simulink model "q_servo_speed_cntrl2"  (R2019a)
settings: Solver=ode4  StartTime=0.0  StopTime=inf  FixedStep=0.002  RelTol=1e-3
values from neighbouring files (symbols this model uses):
  a = 1    [setup_servo_speed_cntrl2.m]
  bsp = 0    [setup_servo_speed_cntrl2.m]
  Kc = 0    [setup_servo_speed_cntrl2.m]
  ki = 0    [setup_servo_speed_cntrl2.m]
  kp = 0    [setup_servo_speed_cntrl2.m]
  T = 1    [setup_servo_speed_cntrl2.m]
undefined symbols (not defined in the file or in its folder): HIL, K_ENC, qc_get_step_size
libraries: quarc_library x6, simulink x2
settings Model: ExtModeTrigDuration=10000  Creator=MLevis  LastModifiedBy=pmartin
settings DataIOCC: ReturnWorkspaceOutputs=off
settings DebuggingCC: UnderspecifiedInitializationDetection=Classic  MergeDetectMultiDrivingBlocksExec=none
settings ModelReferenceCC: PropagateSignalLabelsOutOfModel=off

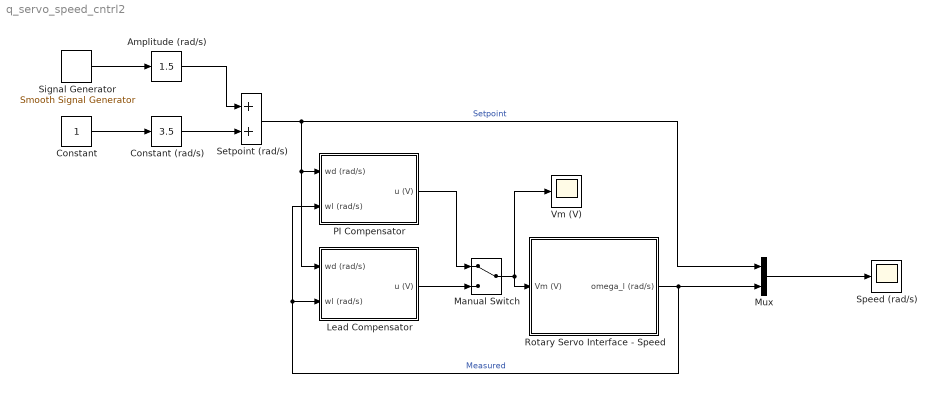
== system q_servo_speed_cntrl2 ==
  Amplitude (rad/s) : simulink/Math Operations/Slider Gain  gain=1.5  low=0  high=10
  "Constant " : Constant
  Constant (rad/s) : simulink/Math Operations/Slider Gain  gain=3.5  low=0  high=10
  Lead Compensator : Subsystem
  Manual Switch : ManualSwitch
  Mux : Mux  Inputs=2
  PI Compensator : Subsystem
  Rotary Servo Interface - Speed : Subsystem
  Setpoint (rad/s) : Sum
  Signal Generator : quarc_library/Sources/Signals/Smooth Signal Generator  signal_type=Square  source=Internal (dialog parameters)  amplitude=1  frequency=0.4  initial_phase=0  sample_time=qc_get_step_size  output_cos=off
      settings: SourceProductName=QUARC Targets
  Speed (rad/s) : Scope
  Vm (V) : Scope
  wires:
  Setpoint (rad/s)/1 -> Mux/1, PI Compensator/1(wd (rad/s)), Lead Compensator/1(wd (rad/s))  "Setpoint"
  Mux/1 -> Speed (rad/s)/1
  Signal Generator/1 -> Amplitude (rad/s)/1
  Amplitude (rad/s)/1 -> Setpoint (rad/s)/1
  "Constant "/1 -> Constant (rad/s)/1
  PI Compensator/1(u (V)) -> Manual Switch/1
  Lead Compensator/1(u (V)) -> Manual Switch/2
  Manual Switch/1 -> Vm (V)/1, Rotary Servo Interface - Speed/1(Vm (V))
  Constant (rad/s)/1 -> Setpoint (rad/s)/2
  Rotary Servo Interface - Speed/1(omega_l (rad/s)) -> Mux/2, Lead Compensator/2(wl (rad/s)), PI Compensator/2(wl (rad/s))  "Measured"

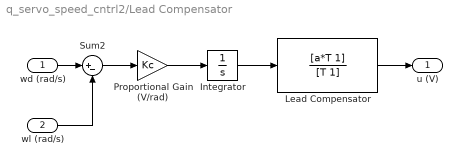
== system q_servo_speed_cntrl2/Lead Compensator ==
  wd (rad/s) : Inport
  wl (rad/s) : Inport  Port=2
  Integrator : Integrator
  Lead Compensator : TransferFcn  Numerator=[a*T 1]  Denominator=[T 1]
  Proportional Gain (V/rad) : Gain  Gain=Kc
  Sum2 : Sum  Inputs=|+-
  u (V) : Outport
  wires:
  wl (rad/s)/1 -> Sum2/2
  wd (rad/s)/1 -> Sum2/1
  Lead Compensator/1 -> u (V)/1
  Sum2/1 -> Proportional Gain (V/rad)/1
  Proportional Gain (V/rad)/1 -> Integrator/1
  Integrator/1 -> Lead Compensator/1

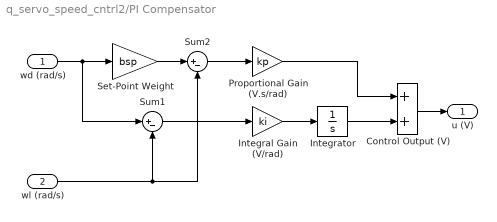
== system q_servo_speed_cntrl2/PI Compensator ==
  wd (rad/s) : Inport
  wl (rad/s) : Inport  Port=2
  Control Output (V) : Sum
  Integral Gain (V/rad) : Gain  Gain=ki
  Integrator : Integrator  UpperSaturationLimit=10  LowerSaturationLimit=-10
  Proportional Gain (V.s/rad) : Gain  Gain=kp
  Set-Point Weight : Gain  Gain=bsp
  Sum1 : Sum  Inputs=|+-
  Sum2 : Sum  Inputs=|+-
  u (V) : Outport
  wires:
  wl (rad/s)/1 -> Sum2/2, Sum1/2
  Control Output (V)/1 -> u (V)/1
  wd (rad/s)/1 -> Sum1/1, Set-Point Weight/1
  Sum2/1 -> Proportional Gain (V.s/rad)/1
  Set-Point Weight/1 -> Sum2/1
  Proportional Gain (V.s/rad)/1 -> Control Output (V)/1
  Integrator/1 -> Control Output (V)/2
  Integral Gain (V/rad)/1 -> Integrator/1
  Sum1/1 -> Integral Gain (V/rad)/1

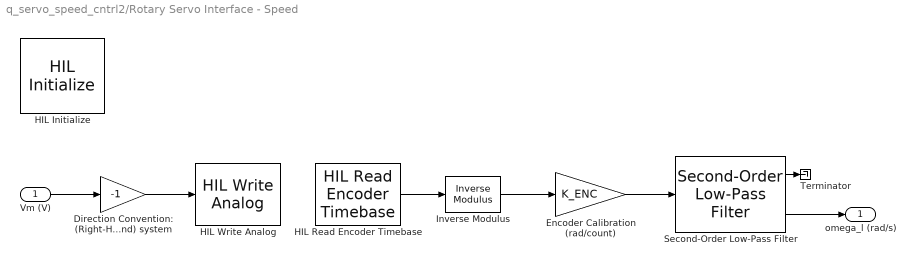
== system q_servo_speed_cntrl2/Rotary Servo Interface - Speed ==
  Vm (V) : Inport
  Direction Convention: (Right-Hand) system : Gain  Gain=-1  SaturateOnIntegerOverflow=on  OutDataTypeStr=Inherit: Same as input  ParamDataTypeStr=Inherit: Same as input
  Encoder Calibration (rad/count) : Gain  Gain=K_ENC  SaturateOnIntegerOverflow=on  OutDataTypeStr=Inherit: Same as input  ParamDataTypeStr=Inherit: Same as input
  HIL Initialize : quarc_library/Data Acquisition/Generic/Configuration/HIL Initialize  object_name=HIL-1  board_type=q8_usb  board_number=0@tcpip://localhost:18940  board_options=update_rate=normal  exclusive=off  active=on  hardware_clocks=[0:2]  clock_modes=[]  initial_clock_frequencies=[]  set_clock_params_at_start=off  set_clock_params_at_switch_in=off  set_clock_frequencies_at_start=off  set_clock_frequencies_at_switch_in=off  analog_input_channels=[0:7]  analog_input_configurations=[]  analog_input_maximums=10  analog_input_minimums=-10  set_analog_input_params_at_start=on  set_analog_input_params_at_switch_in=off  analog_output_channels=[0:7]  analog_output_maximums=10  analog_output_minimums=-10  initial_analog_outputs=[0]  final_analog_outputs=[0]  watchdog_analog_outputs=0  set_analog_output_params_at_start=on  set_analog_output_params_at_switch_in=off  set_analog_outputs_at_start=on  set_analog_outputs_at_switch_in=off  set_analog_outputs_at_terminate=on  set_analog_outputs_at_switch_out=off  set_analog_outputs_on_watchdog=off  digital_input_channels=[]  digital_output_channels=[]  digital_output_configuration=[]  initial_digital_outputs=[1]  final_digital_outputs=[1]  watchdog_digital_outputs=[1]  set_digital_output_params_at_start=off  set_digital_output_params_at_switch_in=off  set_digital_outputs_at_start=on  set_digital_outputs_at_switch_in=off  set_digital_outputs_at_terminate=on  set_digital_outputs_at_switch_out=off  set_digital_outputs_on_watchdog=off  encoder_channels=[0:7]  quadrature=[4]  encoder_filter_frequency=[]  initial_encoder_counts=[0]  set_encoder_params_at_start=on  set_encoder_params_at_switch_in=off  set_encoder_counts_at_start=on  set_encoder_counts_at_switch_in=off  pwm_channels=[0:7]  pwm_modes=0  pwm_frequency=99.532799999999995e6/4095  pwm_configuration=[0]  pwm_alignment=[0]  pwm_polarity=[1]  pwm_leading_deadband=[0]  pwm_trailing_deadband=[0]  initial_pwm_outputs=[0]  final_pwm_outputs=[0]  watchdog_pwm_outputs=[0]  set_pwm_params_at_start=on  set_pwm_params_at_switch_in=off  set_pwm_outputs_at_start=on  set_pwm_outputs_at_switch_in=off  set_pwm_outputs_at_terminate=on  set_pwm_outputs_at_switch_out=off  set_pwm_outputs_on_watchdog=off  other_output_channels=[]  initial_other_outputs=[]  final_other_outputs=[]  watchdog_other_outputs=[]  set_other_outputs_at_start=off  set_other_outputs_at_switch_in=off  set_other_outputs_at_terminate=off  set_other_outputs_at_switch_out=off  set_other_outputs_on_watchdog=off
  HIL Read Encoder Timebase : quarc_library/Data Acquisition/Generic/Timebases/HIL Read Encoder Timebase  object_name=HIL-1  clock=0  channels=0  active=on  vector_output=off  data_type_mode=Inherit via back propagation  data_type=double  overflow_mode=Synchronize (for simulated cards only)  samples_in_buffer=1 + 0 * max(ceil(1/qc_get_step_size), 1)
  HIL Write Analog : quarc_library/Data Acquisition/Generic/Immediate I//O/HIL Write Analog  Tag=unassigned  object_name=HIL-1  channels=0  sample_time=-1  active=on  vector_input=off
  Inverse Modulus : quarc_library/Discontinuities/Inverse Modulus  modulus=2^16  output_derivative=off  output_revolutions=off  max_x=Inf  min_x=-Inf
  Second-Order Low-Pass Filter : quarc_library/Continuous/Second-Order Low-Pass Filter  params_source=Internal (dialog parameters)  input_width=1/0.003  input_zeta=0.9  input_init=0
  Terminator : Terminator
  omega_l (rad/s) : Outport
  wires:
  Direction Convention: (Right-Hand) system/1 -> HIL Write Analog/1
  Vm (V)/1 -> Direction Convention: (Right-Hand) system/1
  HIL Read Encoder Timebase/1 -> Inverse Modulus/1
  Inverse Modulus/1 -> Encoder Calibration (rad/count)/1
  Encoder Calibration (rad/count)/1 -> Second-Order Low-Pass Filter/1
  Second-Order Low-Pass Filter/1 -> Terminator/1
  Second-Order Low-Pass Filter/2 -> omega_l (rad/s)/1
